simulink model "sysgen_grid_pmsm_inv"  (R2016a)
settings: Solver=VariableStepAuto  StartTime=0.0  StopTime=2.5*100e6  RelTol=1e-3
libraries: xbsIndex_r4 x99, powerlib_meascontrol x6
settings Model: Creator=Jorge  LastModifiedBy=Jorge

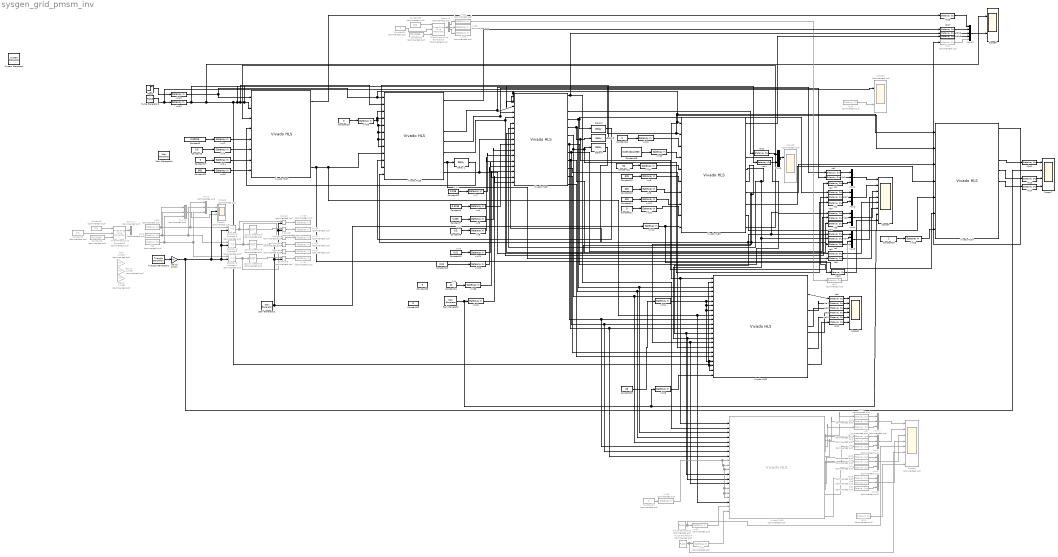
== system sysgen_grid_pmsm_inv ==
  note: 0.04
  note: 0.04
  note: 0.04
  note: 0.04
  " System Generator" : xbsIndex_r4/ System Generator  Tag=genX  xilinxfamily=zynq  part=xc7z020  speed=-1  package=clg400  synthesis_tool=Vivado  clock_wrapper=Clock Enables  directory=./netlist  proj_type=Vivado  Synth_file=Vivado Synthesis Defaults  Impl_file=Vivado Implementation Defaults  testbench=off  simulink_period=1  sysclk_period=10  dcm_input_clock_period=10  incr_netlist=off  trim_vbits=Everywhere in SubSystem  dbl_ovrd=According to Block Masks  core_generation=According to Block Masks  run_coregen=off  deprecated_control=off  eval_field=0  block_type=sysgen
  Constant{10..11,17,29} (4 alike) : Constant  Value=0
  Constant12 : Constant  Value=325
  Constant13 : Constant  Value=325
  Constant14 : Constant  Value=325
  Constant15 : Constant  Value=25
  Constant16 : Constant  Value=0.01
  Constant18 : Constant  Value=(100*1024)/360
  Constant19 : Constant  Value=0.01
  Constant2 : Constant  Value=0.00015
  Constant20 : Constant  Value=0.016
  Constant21 : Constant  Value=800
  Constant22 : Constant  Value=50
  Constant23 : Constant  Value=5
  Constant24 : Constant  Value=11
  Constant26 : Constant
  Constant27 : Constant  Commented=on  Value=0
  Constant28 : Constant  Value=5
  Constant3 : Constant  Value=0.0
  Constant31 : Constant  Commented=on  Value=0
  Constant32 : Constant  Commented=on  Value=50/100e6
  Constant33 : Constant  Commented=on  Value=325
  Constant4 : Constant  Value=0.0016
  Constant5 : Constant  Commented=on  Value=0.0
  Constant6 : Constant  Commented=on  Value=50/100e6
  Constant7 : Constant  Value=0.008
  Constant8 : Constant  Value=0.5
  Constant9 : Constant  Commented=on  Value=0.6
  Delay{1..4} (4 alike) : xbsIndex_r4/Delay  rst=off  infoeditControl=Selection of Reset will increase slice count due to use of real FFs and instead of SRLs  en=off  latency=1  reg_retiming=off  dbl_ovrd=off  block_type=delay
  Demux1 : Demux  Commented=on  Outputs=3
  Demux5 : Demux  Commented=on  Outputs=3
  Gain : Gain  Commented=on  Gain=(1/255)
  Gain1 : Gain  Commented=on  Gain=(1/255)
  Gain2 : Gain  Commented=on  Gain=(1/255)
  Gain3 : Gain  Gain=65535
  Is_a1 : xbsIndex_r4/Gateway Out  Commented=on  inherit_from_input=off  hdl_port=on  rows=1  columns=1  UseAsDAC=off  DACChannel='1'  interface=None  automatic_assignment=on  address_offset=hex2dec('00')  intf_name=''  intf_description=''  timing_constraint=None  locs_specified=off  LOCs={}  io_standard={}  block_type=gatewayout
  Logical Operator3 : Logic  Commented=on  Operator=NOT  AllPortsSameDT=off  OutDataTypeStr=boolean
  Logical Operator4 : Logic  Commented=on  Operator=NOT  AllPortsSameDT=off  OutDataTypeStr=boolean
  Logical Operator5 : Logic  Commented=on  Operator=NOT  AllPortsSameDT=off  OutDataTypeStr=boolean
  Mux1 : Mux  Inputs=3
  Mux{3,7..11} (6 alike) : Mux  Commented=on  Inputs=3
  Mux12 : Mux  Inputs=5
  Mux2 : Mux  Inputs=3
  Mux4 : Mux  Inputs=3
  Mux5 : Mux
  Mux6 : Mux  Inputs=2
  Product{,1..5} (6 alike) : Product  Commented=on
  Pulse Generator2 : DiscretePulseGenerator  PulseType=Time based  Period=80
  Pulse Generator3 : DiscretePulseGenerator  Commented=on  PulseType=Time based  Period=1/(5e3/100e6)
  Pulse Generator4 : DiscretePulseGenerator  Commented=on  PulseType=Time based  Period=1/(2e3/100e6)
  Relational Operator3 : RelationalOperator  Commented=on  OutDataTypeStr=boolean  ZeroCross=off
  Relational Operator4 : RelationalOperator  Commented=on  OutDataTypeStr=boolean  ZeroCross=off
  Relational Operator5 : RelationalOperator  Commented=on  OutDataTypeStr=boolean  ZeroCross=off
  Scope1 : Scope  Commented=on  NumInputPorts=2
  Scope2 : Scope  NumInputPorts=7
  Scope3 : Scope  Commented=on  NumInputPorts=4
  Scope4 : Scope  NumInputPorts=8
  Scope5 : Scope  Commented=on  NumInputPorts=2
  Scope6 : Scope  Commented=on  NumInputPorts=8
  Scope7 : Scope  NumInputPorts=4
  Scope8 : Scope  NumInputPorts=2
  Scope9 : Scope  Commented=on  NumInputPorts=4
  Stair Generator : powerlib_meascontrol/Pulse & Signal Generators/Stair Generator  t=[5000, 12000, 14000000, 70000000]  e=[0, 5, 6, 0]  Ts=0
  Stair Generator1 : powerlib_meascontrol/Pulse & Signal Generators/Stair Generator  t=[10000, 300000000, 350000000]  e=[0, 1, 0]  Ts=0
  Stair Generator2 : powerlib_meascontrol/Pulse & Signal Generators/Stair Generator  t=[5000, 50000000, 60000000]  e=[0, 1, 0]  Ts=0
  Step2 : Step  Time=1e-6  SampleTime=0
  Three-Phase Sine Generator2 : powerlib_meascontrol/Pulse & Signal Generators/Three-Phase Sine Generator  Commented=on  Ts=1
  Three-Phase Sine Generator5 : powerlib_meascontrol/Pulse & Signal Generators/Three-Phase Sine Generator  Commented=on  Ts=1
  Triangle Generator1 : powerlib_meascontrol/Pulse & Signal Generators/Triangle Generator  Freq=3e3/100e6  Phase=90  Ts=1
  Va{1..14} (14 alike) : xbsIndex_r4/Gateway Out  inherit_from_input=off  hdl_port=on  rows=1  columns=1  UseAsDAC=off  DACChannel='1'  interface=None  automatic_assignment=on  address_offset=hex2dec('00')  intf_name=''  intf_description=''  timing_constraint=None  locs_specified=off  LOCs={}  io_standard={}  block_type=gatewayout
  Va{15..21} (7 alike) : xbsIndex_r4/Gateway Out  Commented=on  inherit_from_input=off  hdl_port=on  rows=1  columns=1  UseAsDAC=off  DACChannel='1'  interface=None  automatic_assignment=on  address_offset=hex2dec('00')  intf_name=''  intf_description=''  timing_constraint=None  locs_specified=off  LOCs={}  io_standard={}  block_type=gatewayout
  Vb{1..5,11,13..18} (12 alike) : xbsIndex_r4/Gateway Out  inherit_from_input=off  hdl_port=on  rows=1  columns=1  UseAsDAC=off  DACChannel='1'  interface=None  automatic_assignment=on  address_offset=hex2dec('00')  intf_name=''  intf_description=''  timing_constraint=None  locs_specified=off  LOCs={}  io_standard={}  block_type=gatewayout
  Vb{6..10,12} (6 alike) : xbsIndex_r4/Gateway Out  Commented=on  inherit_from_input=off  hdl_port=on  rows=1  columns=1  UseAsDAC=off  DACChannel='1'  interface=None  automatic_assignment=on  address_offset=hex2dec('00')  intf_name=''  intf_description=''  timing_constraint=None  locs_specified=off  LOCs={}  io_standard={}  block_type=gatewayout
  Vc{1..4} (4 alike) : xbsIndex_r4/Gateway Out  inherit_from_input=off  hdl_port=on  rows=1  columns=1  UseAsDAC=off  DACChannel='1'  interface=None  automatic_assignment=on  address_offset=hex2dec('00')  intf_name=''  intf_description=''  timing_constraint=None  locs_specified=off  LOCs={}  io_standard={}  block_type=gatewayout
  Vc{5..9} (5 alike) : xbsIndex_r4/Gateway Out  Commented=on  inherit_from_input=off  hdl_port=on  rows=1  columns=1  UseAsDAC=off  DACChannel='1'  interface=None  automatic_assignment=on  address_offset=hex2dec('00')  intf_name=''  intf_description=''  timing_constraint=None  locs_specified=off  LOCs={}  io_standard={}  block_type=gatewayout
  Vivado HLS1 : xbsIndex_r4/Vivado HLS  Commented=on  anytable='C:\Users\Jorge\Documents\GitHub\nvHIL\hls\signal_data_extractor_V2\signal_data_extractor_V2_prj\sol_sysgen'  fast_sim=off  display_datatype=on  rate_propagation_method=Simulink system period  model_file_path=''  latency=1  block_type=hls
      settings: infoedit=This block allows including C,C++ and SystemC source files in System Generator for DSP designs.
  Vivado HLS2 : xbsIndex_r4/Vivado HLS  anytable='C:\Users\Jorge\Documents\GitHub\nvHIL\hls\gain_offset_truncation_V2\gain_offset_truncation_prj\sol_sysgen'  fast_sim=off  display_datatype=on  rate_propagation_method=Simulink system period  model_file_path=''  latency=1  block_type=hls
      settings: infoedit=This block allows including C,C++ and SystemC source files in System Generator for DSP designs.
  Vivado HLS3 : xbsIndex_r4/Vivado HLS  anytable='C:\Users\Jorge\Documents\GitHub\nvHIL\hls\grid_V2\grid_prj\sol_sysgen'  fast_sim=off  display_datatype=on  rate_propagation_method=Simulink system period  model_file_path=''  latency=1  block_type=hls
      settings: infoedit=This block allows including C,C++ and SystemC source files in System Generator for DSP designs.
  Vivado HLS4 : xbsIndex_r4/Vivado HLS  anytable='C:\Users\Jorge\Documents\GitHub\nvHIL\hls\3ph_modulator_V2\three_ph_mod_prj\sol_sysgen'  fast_sim=off  display_datatype=on  rate_propagation_method=Simulink system period  model_file_path=''  latency=1  block_type=hls
      settings: infoedit=This block allows including C,C++ and SystemC source files in System Generator for DSP designs.
  Vivado HLS5 : xbsIndex_r4/Vivado HLS  anytable='C:\Users\Jorge\Documents\GitHub\nvHIL\hls\LCL_filter_V2\LCL_filter_prj\sol_sysgen'  fast_sim=off  display_datatype=on  rate_propagation_method=Simulink system period  model_file_path=''  latency=1  block_type=hls
      settings: infoedit=This block allows including C,C++ and SystemC source files in System Generator for DSP designs.
  Vivado HLS6 : xbsIndex_r4/Vivado HLS  anytable='C:\Users\Jorge\Documents\GitHub\nvHIL\hls\grid_3ph_inv_V2\grid_3ph_bridge_prj\sol_sysgen'  fast_sim=off  display_datatype=on  rate_propagation_method=Simulink system period  model_file_path=''  latency=1  block_type=hls
      settings: infoedit=This block allows including C,C++ and SystemC source files in System Generator for DSP designs.
  Vivado HLS7 : xbsIndex_r4/Vivado HLS  anytable='C:\Users\Jorge\Documents\GitHub\nvHIL\hls\DC_bus_V2\dc_bus_prj\sol_sysgen'  fast_sim=off  display_datatype=on  rate_propagation_method=Simulink system period  model_file_path=''  latency=1  block_type=hls
      settings: infoedit=This block allows including C,C++ and SystemC source files in System Generator for DSP designs.
  xin10 : xbsIndex_r4/Gateway In  gui_display_data_type=Boolean  arith_type=Boolean  n_bits=2  bin_pt=1  preci_type=Single  exp_width=8  frac_width=24  rows=1  columns=1  quantization="Round  (unbiased: +/- Inf)"  overflow=Saturate  period=1  UseAsADC=off  ADCChannel='1'  interface=None  automatic_assignment=on  address_offset=hex2dec('00')  intf_name=''  intf_description=''  default_value=0  timing_constraint=None  locs_specified=off  LOCs={}  io_standard={}  inherit_from_input=off  hdl_port=on  dbl_ovrd=off  block_type=gatewayin
  xin11 : xbsIndex_r4/Gateway In  gui_display_data_type=Boolean  arith_type=Boolean  n_bits=25  bin_pt=9  preci_type=Single  exp_width=8  frac_width=24  rows=1  columns=1  quantization="Round  (unbiased: +/- Inf)"  overflow=Saturate  period=1  UseAsADC=off  ADCChannel='1'  interface=None  automatic_assignment=on  address_offset=hex2dec('00')  intf_name=''  intf_description=''  default_value=0  timing_constraint=None  locs_specified=off  LOCs={}  io_standard={}  inherit_from_input=off  hdl_port=on  dbl_ovrd=off  block_type=gatewayin
  xin12 : xbsIndex_r4/Gateway In  gui_display_data_type=Floating-point  arith_type=Floating-point  n_bits=25  bin_pt=9  preci_type=Single  exp_width=8  frac_width=24  rows=1  columns=1  quantization="Round  (unbiased: +/- Inf)"  overflow=Saturate  period=1  UseAsADC=off  ADCChannel='1'  interface=None  automatic_assignment=on  address_offset=hex2dec('00')  intf_name=''  intf_description=''  default_value=0  timing_constraint=None  locs_specified=off  LOCs={}  io_standard={}  inherit_from_input=off  hdl_port=on  dbl_ovrd=off  block_type=gatewayin
  xin{13..18} (6 alike) : xbsIndex_r4/Gateway In  Commented=on  gui_display_data_type=Boolean  arith_type=Boolean  n_bits=18  bin_pt=6  preci_type=Single  exp_width=8  frac_width=24  rows=1  columns=1  quantization="Round  (unbiased: +/- Inf)"  overflow=Saturate  period=1  UseAsADC=off  ADCChannel='1'  interface=None  automatic_assignment=on  address_offset=hex2dec('00')  intf_name=''  intf_description=''  default_value=0  timing_constraint=None  locs_specified=off  LOCs={}  io_standard={}  inherit_from_input=off  hdl_port=on  dbl_ovrd=off  block_type=gatewayin
  xin19 : xbsIndex_r4/Gateway In  gui_display_data_type=Boolean  arith_type=Boolean  n_bits=16  bin_pt=10  preci_type=Single  exp_width=8  frac_width=24  rows=1  columns=1  quantization="Round  (unbiased: +/- Inf)"  overflow=Saturate  period=1  UseAsADC=off  ADCChannel='1'  interface=None  automatic_assignment=on  address_offset=hex2dec('00')  intf_name=''  intf_description=''  default_value=0  timing_constraint=None  locs_specified=off  LOCs={}  io_standard={}  inherit_from_input=off  hdl_port=on  dbl_ovrd=off  block_type=gatewayin
  xin2 : xbsIndex_r4/Gateway In  gui_display_data_type=Floating-point  arith_type=Floating-point  n_bits=19  bin_pt=18  preci_type=Single  exp_width=8  frac_width=24  rows=1  columns=1  quantization="Round  (unbiased: +/- Inf)"  overflow=Saturate  period=1  UseAsADC=off  ADCChannel='1'  interface=None  automatic_assignment=on  address_offset=hex2dec('00')  intf_name=''  intf_description=''  default_value=0  timing_constraint=None  locs_specified=off  LOCs={}  io_standard={}  inherit_from_input=off  hdl_port=on  dbl_ovrd=off  block_type=gatewayin
  xin20 : xbsIndex_r4/Gateway In  gui_display_data_type=Boolean  arith_type=Boolean  n_bits=16  bin_pt=10  preci_type=Single  exp_width=8  frac_width=24  rows=1  columns=1  quantization="Round  (unbiased: +/- Inf)"  overflow=Saturate  period=1  UseAsADC=off  ADCChannel='1'  interface=None  automatic_assignment=on  address_offset=hex2dec('00')  intf_name=''  intf_description=''  default_value=0  timing_constraint=None  locs_specified=off  LOCs={}  io_standard={}  inherit_from_input=off  hdl_port=on  dbl_ovrd=off  block_type=gatewayin
  xin21 : xbsIndex_r4/Gateway In  gui_display_data_type=Floating-point  arith_type=Floating-point  n_bits=30  bin_pt=7  preci_type=Single  exp_width=8  frac_width=24  rows=1  columns=1  quantization="Round  (unbiased: +/- Inf)"  overflow=Saturate  period=1  UseAsADC=off  ADCChannel='1'  interface=None  automatic_assignment=on  address_offset=hex2dec('00')  intf_name=''  intf_description=''  default_value=0  timing_constraint=None  locs_specified=off  LOCs={}  io_standard={}  inherit_from_input=off  hdl_port=on  dbl_ovrd=off  block_type=gatewayin
  xin22 : xbsIndex_r4/Gateway In  gui_display_data_type=Boolean  arith_type=Boolean  n_bits=25  bin_pt=9  preci_type=Single  exp_width=8  frac_width=24  rows=1  columns=1  quantization="Round  (unbiased: +/- Inf)"  overflow=Saturate  period=1  UseAsADC=off  ADCChannel='1'  interface=None  automatic_assignment=on  address_offset=hex2dec('00')  intf_name=''  intf_description=''  default_value=0  timing_constraint=None  locs_specified=off  LOCs={}  io_standard={}  inherit_from_input=off  hdl_port=on  dbl_ovrd=off  block_type=gatewayin
  xin23 : xbsIndex_r4/Gateway In  gui_display_data_type=Floating-point  arith_type=Floating-point  n_bits=32  bin_pt=0  preci_type=Single  exp_width=8  frac_width=24  rows=1  columns=1  quantization="Round  (unbiased: +/- Inf)"  overflow=Saturate  period=1  UseAsADC=off  ADCChannel='1'  interface=None  automatic_assignment=on  address_offset=hex2dec('00')  intf_name=''  intf_description=''  default_value=0  timing_constraint=None  locs_specified=off  LOCs={}  io_standard={}  inherit_from_input=off  hdl_port=on  dbl_ovrd=off  block_type=gatewayin
  xin24 : xbsIndex_r4/Gateway In  gui_display_data_type=Boolean  arith_type=Boolean  n_bits=2  bin_pt=1  preci_type=Single  exp_width=8  frac_width=24  rows=1  columns=1  quantization="Round  (unbiased: +/- Inf)"  overflow=Saturate  period=1  UseAsADC=off  ADCChannel='1'  interface=None  automatic_assignment=on  address_offset=hex2dec('00')  intf_name=''  intf_description=''  default_value=0  timing_constraint=None  locs_specified=off  LOCs={}  io_standard={}  inherit_from_input=off  hdl_port=on  dbl_ovrd=off  block_type=gatewayin
  xin25 : xbsIndex_r4/Gateway In  gui_display_data_type=Floating-point  arith_type=Floating-point  n_bits=30  bin_pt=7  preci_type=Single  exp_width=8  frac_width=24  rows=1  columns=1  quantization="Round  (unbiased: +/- Inf)"  overflow=Saturate  period=1  UseAsADC=off  ADCChannel='1'  interface=None  automatic_assignment=on  address_offset=hex2dec('00')  intf_name=''  intf_description=''  default_value=0  timing_constraint=None  locs_specified=off  LOCs={}  io_standard={}  inherit_from_input=off  hdl_port=on  dbl_ovrd=off  block_type=gatewayin
  xin26 : xbsIndex_r4/Gateway In  gui_display_data_type=Floating-point  arith_type=Floating-point  n_bits=18  bin_pt=6  preci_type=Single  exp_width=8  frac_width=24  rows=1  columns=1  quantization="Round  (unbiased: +/- Inf)"  overflow=Saturate  period=1  UseAsADC=off  ADCChannel='1'  interface=None  automatic_assignment=on  address_offset=hex2dec('00')  intf_name=''  intf_description=''  default_value=0  timing_constraint=None  locs_specified=off  LOCs={}  io_standard={}  inherit_from_input=off  hdl_port=on  dbl_ovrd=off  block_type=gatewayin
  xin27 : xbsIndex_r4/Gateway In  gui_display_data_type=Fixed-point  arith_type="Signed  (2's comp)"  n_bits=32  bin_pt=0  preci_type=Single  exp_width=8  frac_width=24  rows=1  columns=1  quantization="Round  (unbiased: +/- Inf)"  overflow=Saturate  period=1  UseAsADC=off  ADCChannel='1'  interface=None  automatic_assignment=on  address_offset=hex2dec('00')  intf_name=''  intf_description=''  default_value=0  timing_constraint=None  locs_specified=off  LOCs={}  io_standard={}  inherit_from_input=off  hdl_port=on  dbl_ovrd=off  block_type=gatewayin
  xin28 : xbsIndex_r4/Gateway In  gui_display_data_type=Fixed-point  arith_type=Unsigned  n_bits=3  bin_pt=0  preci_type=Single  exp_width=8  frac_width=24  rows=1  columns=1  quantization="Round  (unbiased: +/- Inf)"  overflow=Saturate  period=1  UseAsADC=off  ADCChannel='1'  interface=None  automatic_assignment=on  address_offset=hex2dec('00')  intf_name=''  intf_description=''  default_value=0  timing_constraint=None  locs_specified=off  LOCs={}  io_standard={}  inherit_from_input=off  hdl_port=on  dbl_ovrd=off  block_type=gatewayin
  xin29 : xbsIndex_r4/Gateway In  gui_display_data_type=Fixed-point  arith_type="Signed  (2's comp)"  n_bits=12  bin_pt=0  preci_type=Single  exp_width=8  frac_width=24  rows=1  columns=1  quantization="Round  (unbiased: +/- Inf)"  overflow=Saturate  period=1  UseAsADC=off  ADCChannel='1'  interface=None  automatic_assignment=on  address_offset=hex2dec('00')  intf_name=''  intf_description=''  default_value=0  timing_constraint=None  locs_specified=off  LOCs={}  io_standard={}  inherit_from_input=off  hdl_port=on  dbl_ovrd=off  block_type=gatewayin
  xin3 : xbsIndex_r4/Gateway In  gui_display_data_type=Boolean  arith_type=Boolean  n_bits=2  bin_pt=1  preci_type=Single  exp_width=8  frac_width=24  rows=1  columns=1  quantization="Round  (unbiased: +/- Inf)"  overflow=Saturate  period=1  UseAsADC=off  ADCChannel='1'  interface=None  automatic_assignment=on  address_offset=hex2dec('00')  intf_name=''  intf_description=''  default_value=0  timing_constraint=None  locs_specified=off  LOCs={}  io_standard={}  inherit_from_input=off  hdl_port=on  dbl_ovrd=off  block_type=gatewayin
  xin30 : xbsIndex_r4/Gateway In  Commented=on  gui_display_data_type=Fixed-point  arith_type="Signed  (2's comp)"  n_bits=25  bin_pt=9  preci_type=Single  exp_width=8  frac_width=24  rows=1  columns=1  quantization="Round  (unbiased: +/- Inf)"  overflow=Saturate  period=1  UseAsADC=off  ADCChannel='1'  interface=None  automatic_assignment=on  address_offset=hex2dec('00')  intf_name=''  intf_description=''  default_value=0  timing_constraint=None  locs_specified=off  LOCs={}  io_standard={}  inherit_from_input=off  hdl_port=on  dbl_ovrd=off  block_type=gatewayin
  xin31 : xbsIndex_r4/Gateway In  Commented=on  gui_display_data_type=Boolean  arith_type=Boolean  n_bits=25  bin_pt=9  preci_type=Single  exp_width=8  frac_width=24  rows=1  columns=1  quantization="Round  (unbiased: +/- Inf)"  overflow=Saturate  period=1  UseAsADC=off  ADCChannel='1'  interface=None  automatic_assignment=on  address_offset=hex2dec('00')  intf_name=''  intf_description=''  default_value=0  timing_constraint=None  locs_specified=off  LOCs={}  io_standard={}  inherit_from_input=off  hdl_port=on  dbl_ovrd=off  block_type=gatewayin
  xin32 : xbsIndex_r4/Gateway In  Commented=on  gui_display_data_type=Boolean  arith_type=Boolean  n_bits=25  bin_pt=9  preci_type=Single  exp_width=8  frac_width=24  rows=1  columns=1  quantization="Round  (unbiased: +/- Inf)"  overflow=Saturate  period=1  UseAsADC=off  ADCChannel='1'  interface=None  automatic_assignment=on  address_offset=hex2dec('00')  intf_name=''  intf_description=''  default_value=0  timing_constraint=None  locs_specified=off  LOCs={}  io_standard={}  inherit_from_input=off  hdl_port=on  dbl_ovrd=off  block_type=gatewayin
  xin33 : xbsIndex_r4/Gateway In  gui_display_data_type=Boolean  arith_type=Boolean  n_bits=32  bin_pt=20  preci_type=Single  exp_width=8  frac_width=24  rows=1  columns=1  quantization="Round  (unbiased: +/- Inf)"  overflow=Saturate  period=1  UseAsADC=off  ADCChannel='1'  interface=None  automatic_assignment=on  address_offset=hex2dec('00')  intf_name=''  intf_description=''  default_value=0  timing_constraint=None  locs_specified=off  LOCs={}  io_standard={}  inherit_from_input=off  hdl_port=on  dbl_ovrd=off  block_type=gatewayin
  xin34 : xbsIndex_r4/Gateway In  gui_display_data_type=Floating-point  arith_type=Floating-point  n_bits=32  bin_pt=20  preci_type=Single  exp_width=8  frac_width=24  rows=1  columns=1  quantization="Round  (unbiased: +/- Inf)"  overflow=Saturate  period=1  UseAsADC=off  ADCChannel='1'  interface=None  automatic_assignment=on  address_offset=hex2dec('00')  intf_name=''  intf_description=''  default_value=0  timing_constraint=None  locs_specified=off  LOCs={}  io_standard={}  inherit_from_input=off  hdl_port=on  dbl_ovrd=off  block_type=gatewayin
  xin36 : xbsIndex_r4/Gateway In  gui_display_data_type=Floating-point  arith_type=Floating-point  n_bits=32  bin_pt=7  preci_type=Single  exp_width=8  frac_width=24  rows=1  columns=1  quantization="Round  (unbiased: +/- Inf)"  overflow=Saturate  period=1  UseAsADC=off  ADCChannel='1'  interface=None  automatic_assignment=on  address_offset=hex2dec('00')  intf_name=''  intf_description=''  default_value=0  timing_constraint=None  locs_specified=off  LOCs={}  io_standard={}  inherit_from_input=off  hdl_port=on  dbl_ovrd=off  block_type=gatewayin
  xin37 : xbsIndex_r4/Gateway In  Commented=on  gui_display_data_type=Fixed-point  arith_type="Signed  (2's comp)"  n_bits=32  bin_pt=20  preci_type=Single  exp_width=8  frac_width=24  rows=1  columns=1  quantization="Round  (unbiased: +/- Inf)"  overflow=Saturate  period=1  UseAsADC=off  ADCChannel='1'  interface=None  automatic_assignment=on  address_offset=hex2dec('00')  intf_name=''  intf_description=''  default_value=0  timing_constraint=None  locs_specified=off  LOCs={}  io_standard={}  inherit_from_input=off  hdl_port=on  dbl_ovrd=off  block_type=gatewayin
  xin38 : xbsIndex_r4/Gateway In  Commented=on  gui_display_data_type=Fixed-point  arith_type="Signed  (2's comp)"  n_bits=32  bin_pt=20  preci_type=Single  exp_width=8  frac_width=24  rows=1  columns=1  quantization="Round  (unbiased: +/- Inf)"  overflow=Saturate  period=1  UseAsADC=off  ADCChannel='1'  interface=None  automatic_assignment=on  address_offset=hex2dec('00')  intf_name=''  intf_description=''  default_value=0  timing_constraint=None  locs_specified=off  LOCs={}  io_standard={}  inherit_from_input=off  hdl_port=on  dbl_ovrd=off  block_type=gatewayin
  xin39 : xbsIndex_r4/Gateway In  Commented=on  gui_display_data_type=Fixed-point  arith_type="Signed  (2's comp)"  n_bits=32  bin_pt=20  preci_type=Single  exp_width=8  frac_width=24  rows=1  columns=1  quantization="Round  (unbiased: +/- Inf)"  overflow=Saturate  period=1  UseAsADC=off  ADCChannel='1'  interface=None  automatic_assignment=on  address_offset=hex2dec('00')  intf_name=''  intf_description=''  default_value=0  timing_constraint=None  locs_specified=off  LOCs={}  io_standard={}  inherit_from_input=off  hdl_port=on  dbl_ovrd=off  block_type=gatewayin
  xin4 : xbsIndex_r4/Gateway In  gui_display_data_type=Floating-point  arith_type=Floating-point  n_bits=16  bin_pt=15  preci_type=Single  exp_width=8  frac_width=24  rows=1  columns=1  quantization="Round  (unbiased: +/- Inf)"  overflow=Saturate  period=1  UseAsADC=off  ADCChannel='1'  interface=None  automatic_assignment=on  address_offset=hex2dec('00')  intf_name=''  intf_description=''  default_value=0  timing_constraint=None  locs_specified=off  LOCs={}  io_standard={}  inherit_from_input=off  hdl_port=on  dbl_ovrd=off  block_type=gatewayin
  xin40 : xbsIndex_r4/Gateway In  gui_display_data_type=Fixed-point  arith_type="Signed  (2's comp)"  n_bits=5  bin_pt=0  preci_type=Single  exp_width=8  frac_width=24  rows=1  columns=1  quantization="Round  (unbiased: +/- Inf)"  overflow=Saturate  period=1  UseAsADC=off  ADCChannel='1'  interface=None  automatic_assignment=on  address_offset=hex2dec('00')  intf_name=''  intf_description=''  default_value=0  timing_constraint=None  locs_specified=off  LOCs={}  io_standard={}  inherit_from_input=off  hdl_port=on  dbl_ovrd=off  block_type=gatewayin
  xin5 : xbsIndex_r4/Gateway In  gui_display_data_type=Floating-point  arith_type=Floating-point  n_bits=16  bin_pt=15  preci_type=Single  exp_width=8  frac_width=24  rows=1  columns=1  quantization="Round  (unbiased: +/- Inf)"  overflow=Saturate  period=1  UseAsADC=off  ADCChannel='1'  interface=None  automatic_assignment=on  address_offset=hex2dec('00')  intf_name=''  intf_description=''  default_value=0  timing_constraint=None  locs_specified=off  LOCs={}  io_standard={}  inherit_from_input=off  hdl_port=on  dbl_ovrd=off  block_type=gatewayin
  xin6 : xbsIndex_r4/Gateway In  gui_display_data_type=Floating-point  arith_type=Floating-point  n_bits=31  bin_pt=10  preci_type=Single  exp_width=8  frac_width=24  rows=1  columns=1  quantization="Round  (unbiased: +/- Inf)"  overflow=Saturate  period=1  UseAsADC=off  ADCChannel='1'  interface=None  automatic_assignment=on  address_offset=hex2dec('00')  intf_name=''  intf_description=''  default_value=0  timing_constraint=None  locs_specified=off  LOCs={}  io_standard={}  inherit_from_input=off  hdl_port=on  dbl_ovrd=off  block_type=gatewayin
  xin7 : xbsIndex_r4/Gateway In  gui_display_data_type=Floating-point  arith_type=Floating-point  n_bits=16  bin_pt=15  preci_type=Single  exp_width=8  frac_width=24  rows=1  columns=1  quantization="Round  (unbiased: +/- Inf)"  overflow=Saturate  period=1  UseAsADC=off  ADCChannel='1'  interface=None  automatic_assignment=on  address_offset=hex2dec('00')  intf_name=''  intf_description=''  default_value=0  timing_constraint=None  locs_specified=off  LOCs={}  io_standard={}  inherit_from_input=off  hdl_port=on  dbl_ovrd=off  block_type=gatewayin
  xin8 : xbsIndex_r4/Gateway In  gui_display_data_type=Floating-point  arith_type=Floating-point  n_bits=25  bin_pt=9  preci_type=Single  exp_width=8  frac_width=24  rows=1  columns=1  quantization="Round  (unbiased: +/- Inf)"  overflow=Saturate  period=1  UseAsADC=off  ADCChannel='1'  interface=None  automatic_assignment=on  address_offset=hex2dec('00')  intf_name=''  intf_description=''  default_value=0  timing_constraint=None  locs_specified=off  LOCs={}  io_standard={}  inherit_from_input=off  hdl_port=on  dbl_ovrd=off  block_type=gatewayin
  xin9 : xbsIndex_r4/Gateway In  gui_display_data_type=Floating-point  arith_type=Floating-point  n_bits=25  bin_pt=9  preci_type=Single  exp_width=8  frac_width=24  rows=1  columns=1  quantization="Round  (unbiased: +/- Inf)"  overflow=Saturate  period=1  UseAsADC=off  ADCChannel='1'  interface=None  automatic_assignment=on  address_offset=hex2dec('00')  intf_name=''  intf_description=''  default_value=0  timing_constraint=None  locs_specified=off  LOCs={}  io_standard={}  inherit_from_input=off  hdl_port=on  dbl_ovrd=off  block_type=gatewayin
  wires:
  Is_a1/1 -> Scope1/2
  Step2/1 -> xin19/1
  Pulse Generator2/1 -> Scope1/1, xin20/1
  xin19/1 -> Vivado HLS7/1, Vivado HLS1/1, Vivado HLS2/1, Vivado HLS3/1, Vivado HLS4/1, Vivado HLS5/1, Vivado HLS6/1
  xin20/1 -> Va14/1, Scope8/1, Vivado HLS2/2, Vivado HLS4/2, Vivado HLS3/2, Vivado HLS6/2, Vivado HLS5/2, Vivado HLS7/2
  Constant2/1 -> xin2/1
  xin2/1 -> Vivado HLS7/5
  Constant3/1 -> xin3/1
  xin3/1 -> Vivado HLS7/6
  Vivado HLS5/4 -> Vivado HLS1/3, Vivado HLS2/3, Delay2/1, Va2/1
  Vivado HLS5/5 -> Vivado HLS1/4, Vivado HLS2/4, Vb2/1, Delay3/1
  Vivado HLS5/6 -> Vivado HLS1/5, Vivado HLS2/5, Delay4/1, Vc2/1
  Constant4/1 -> xin4/1
  Constant7/1 -> xin5/1
  Constant8/1 -> xin6/1
  xin4/1 -> Vivado HLS5/10
  xin5/1 -> Vivado HLS5/11
  Vivado HLS6/8 -> Vivado HLS5/9, Va5/1
  Vivado HLS6/4 -> Va1/1, Vivado HLS5/3
  Vivado HLS6/5 -> Vb1/1, Vivado HLS5/4
  Vivado HLS6/6 -> Vc1/1, Vivado HLS5/5
  Va1/1 -> Mux1/1
  Vb1/1 -> Mux1/2
  Vc1/1 -> Mux1/3
  Va2/1 -> Mux2/1
  Vb2/1 -> Mux2/2
  Vc2/1 -> Mux2/3
  Delay2/1 -> Vivado HLS6/10
  Delay3/1 -> Vivado HLS6/11
  Delay4/1 -> Vivado HLS6/12
  Va3/1 -> Mux4/1
  Vb3/1 -> Mux4/2
  Vc3/1 -> Mux4/3
  Va4/1 -> Mux5/1
  Vb4/1 -> Mux5/2
  Vc4/1 -> Mux5/3
  Constant16/1 -> xin21/1
  Constant12/1 -> xin8/1
  Constant13/1 -> xin9/1
  Constant14/1 -> xin12/1
  Constant18/1 -> xin23/1
  Constant17/1 -> xin24/1
  xin24/1 -> Vivado HLS7/7
  Constant20/1 -> xin7/1
  xin7/1 -> Vivado HLS5/12
  xin6/1 -> Vivado HLS5/13
  xin21/1 -> Vivado HLS5/14
  xin25/1 -> Vivado HLS5/15
  Va5/1 -> Scope4/5
  Vb5/1 -> Scope4/6
  Constant21/1 -> xin26/1
  xin26/1 -> Vivado HLS7/8
  xin23/1 -> Vivado HLS3/4
  xin8/1 -> Vivado HLS3/6
  xin9/1 -> Vivado HLS3/7
  xin12/1 -> Vivado HLS3/8
  xin10/1 -> Vivado HLS3/3
  Constant22/1 -> xin27/1
  xin27/1 -> Vivado HLS3/5
  Vivado HLS5/7 -> Vivado HLS1/6, Vivado HLS2/10, Va3/1
  Vivado HLS5/8 -> Vivado HLS1/7, Vivado HLS2/11, Vb3/1
  Vivado HLS5/9 -> Vivado HLS1/8, Vivado HLS2/12, Vc3/1
  Mux1/1 -> Scope4/1
  Mux2/1 -> Scope4/2
  Mux4/1 -> Scope4/3
  Mux5/1 -> Scope4/4
  Constant10/1 -> xin10/1
  Constant19/1 -> xin25/1
  Vivado HLS7/4 -> Vivado HLS1/18, Vivado HLS2/9, Vivado HLS6/9, Va13/1
  Vivado HLS2/4 -> Va6/1
  Vivado HLS2/7 -> Va7/1
  Vivado HLS2/10 -> Va8/1
  Vivado HLS2/11 -> Va9/1
  Vivado HLS2/14 -> Va10/1
  Vivado HLS2/17 -> Va11/1
  Va6/1 -> Scope2/1
  Va7/1 -> Scope2/2
  Va8/1 -> Scope2/3
  Va9/1 -> Scope2/4
  Va10/1 -> Scope2/5
  Va11/1 -> Scope2/6
  Vivado HLS3/6 -> Vivado HLS5/8, Vivado HLS1/14, Vivado HLS2/15, Vc4/1
  Vivado HLS3/5 -> Vivado HLS5/7, Vivado HLS1/13, Vivado HLS2/14, Vb4/1
  Vivado HLS3/4 -> Vivado HLS1/12, Vivado HLS2/13, Vivado HLS5/6, Va4/1
  Va12/1 -> Mux6/1
  Mux6/1 -> Scope5/1
  Constant11/1 -> xin22/1
  xin22/1 -> Vivado HLS3/9
  Constant15/1 -> xin34/1
  xin28/1 -> Vivado HLS2/22
  xin34/1 -> Vivado HLS2/21, Vivado HLS2/20, Vivado HLS2/19, Vivado HLS2/8, Vivado HLS2/7, Vivado HLS2/6
  Stair Generator/1 -> xin28/1, Scope4/7, xin40/1
  Vivado HLS5/1 -> Vb16/1, Vivado HLS1/2
  Constant24/1 -> xin36/1
  xin36/1 -> Vivado HLS5/16
  xin40/1 -> Vivado HLS5/17
  Vivado HLS5/10 -> Vivado HLS2/16
  Vivado HLS5/11 -> Vivado HLS2/17
  Vivado HLS5/12 -> Vivado HLS2/18
  Va13/1 -> Scope4/8
  Triangle Generator1/1 -> Gain3/1
  Relational Operator3/1 -> Product/1, Logical Operator3/1
  Constant6/1 -> Three-Phase Sine Generator2/3
  Constant9/1 -> Three-Phase Sine Generator2/1
  Mux3/1 -> Scope3/1
  Constant5/1 -> Three-Phase Sine Generator2/2
  Relational Operator4/1 -> Product4/1, Logical Operator5/1
  Relational Operator5/1 -> Product2/1, Logical Operator4/1
  Vivado HLS5/3 -> Va12/1
  Va14/1 -> Mux6/2
  Constant27/1 -> xin30/1
  xin30/1 -> Vivado HLS1/17, Vivado HLS1/16, Vivado HLS1/15, Vivado HLS1/11, Vivado HLS1/10, Vivado HLS1/9
  xin31/1 -> Vivado HLS1/19
  xin32/1 -> Vivado HLS1/20
  Va15/1 -> Mux7/1
  Vb6/1 -> Mux7/2
  Vc5/1 -> Mux7/3
  Va17/1 -> Mux8/1
  Vb7/1 -> Mux8/2
  Vc6/1 -> Mux8/3
  Va18/1 -> Mux9/1
  Vb8/1 -> Mux9/2
  Vc7/1 -> Mux9/3
  Va19/1 -> Mux10/1
  Vb9/1 -> Mux10/2
  Vc8/1 -> Mux10/3
  Pulse Generator3/1 -> Scope6/5, xin31/1
  Pulse Generator4/1 -> Scope6/6, xin32/1
  Mux7/1 -> Scope6/1
  Mux8/1 -> Scope6/2
  Mux9/1 -> Scope6/3
  Mux10/1 -> Scope6/4
  Va16/1 -> Scope6/8
  Vivado HLS1/4 -> Va15/1
  Vivado HLS1/5 -> Vb6/1
  Vivado HLS1/6 -> Vc5/1
  Vivado HLS1/7 -> Va17/1
  Vivado HLS1/8 -> Vb7/1
  Vivado HLS1/9 -> Vc6/1
  Vivado HLS1/13 -> Va18/1
  Vivado HLS1/14 -> Vb8/1
  Vivado HLS1/15 -> Vc7/1
  Vivado HLS1/19 -> Va19/1
  Vivado HLS6/7 -> Delay1/1, Vb5/1
  Delay1/1 -> Vivado HLS7/4
  Constant32/1 -> Three-Phase Sine Generator5/3
  Constant33/1 -> Three-Phase Sine Generator5/1
  Constant31/1 -> Three-Phase Sine Generator5/2
  Three-Phase Sine Generator5/1 -> Demux5/1
  Demux5/2 -> xin38/1
  Demux5/1 -> xin37/1
  Demux5/3 -> xin39/1
  xin37/1 -> Va20/1
  Va20/1 -> Mux5/4
  Three-Phase Sine Generator2/1 -> Demux1/1
  Stair Generator2/1 -> Product5/2, Product4/2, Product3/2, Product2/2, Product1/2, Product/2, xin11/1
  xin11/1 -> Vivado HLS4/6, Vivado HLS3/10
  Product/1 -> xin15/1
  Product1/1 -> xin16/1
  Logical Operator3/1 -> Product1/1
  Product2/1 -> xin17/1
  Logical Operator4/1 -> Product3/1
  Product3/1 -> xin18/1
  Product4/1 -> xin13/1
  Logical Operator5/1 -> Product5/1
  Product5/1 -> xin14/1
  Mux11/1 -> Scope3/3
  Vc9/1 -> Relational Operator4/1, Mux3/3, Mux11/3
  Vb10/1 -> Mux3/2, Relational Operator5/1, Mux11/2
  Va21/1 -> Mux3/1, Relational Operator3/1, Mux11/1
  Constant26/1 -> xin29/1
  xin29/1 -> Vivado HLS4/7
  Vivado HLS4/4 -> Vb11/1
  Vb11/1 -> Scope7/1
  Gain3/1 -> Scope7/2, Scope3/2, Relational Operator4/2, Relational Operator5/2, Relational Operator3/2
  Vb13/1 -> Scope7/3
  Vivado HLS4/5 -> Vb13/1
  Vb14/1 -> Scope7/4
  Mux12/1 -> Scope8/2
  Vivado HLS4/1 -> Vb12/1
  Vivado HLS3/1 -> Vb15/1
  Vivado HLS6/1 -> Vb17/1
  Vivado HLS7/1 -> Vb18/1
  Vb12/1 -> Mux12/5
  Vb15/1 -> Mux12/4
  Vb16/1 -> Mux12/3
  Vb17/1 -> Mux12/2
  Vb18/1 -> Mux12/1
  Vivado HLS3/10 -> Vivado HLS7/3
  Constant29/1 -> xin33/1
  xin33/1 -> Vivado HLS6/4, Vivado HLS6/3, Vivado HLS6/8, Vivado HLS6/7, Vivado HLS6/6, Vivado HLS6/5
  Vivado HLS3/7 -> Vivado HLS4/3
  Vivado HLS3/8 -> Vivado HLS4/4
  Vivado HLS3/9 -> Vivado HLS4/5
  Vivado HLS4/6 -> Vb14/1
